simulink model "dvanaestaNedeljaPrimeri"  (R2018a)
settings: Solver=ode4  StartTime=0.0  StopTime=10  FixedStep=.01  RelTol=1e-3
values from neighbouring files (symbols this model uses):
  co = 10    [konstante.m]
  cp = [0 2 8]    [konstante.m]
  m = 1    [konstante.m]
undefined symbols (not defined in the file or in its folder): b
libraries: simulink x1
settings Model: Creator=Teodor  LastModifiedBy=Teodor

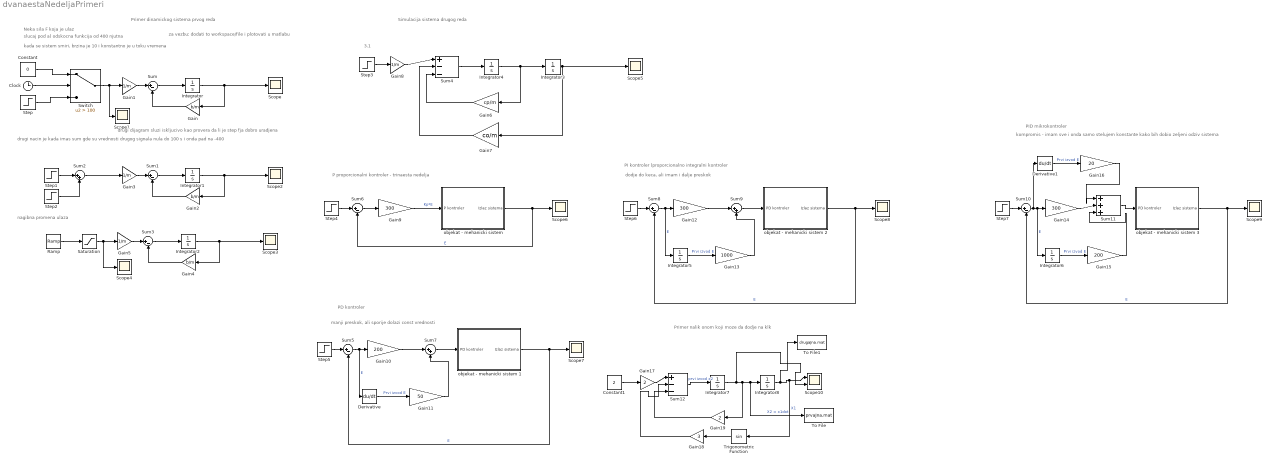
== system dvanaestaNedeljaPrimeri ==
  note: Primer nalik onom koji moze da dodje na klk
  note: kompromis - imam sve i onda samo stelujem konstante kako bih dobio zeljeni odziv sistema
  note: PID mikrokontroler
  note: dodje do keca, ali imam i dalje preskok
  note: PI kontroler (proporcionalno integralni kontroler
  note: manji preskok, ali sporije dolazi const vrednosti
  note: PD kontroler
  note: 3.1
  note: Simulacija sistema drugog reda
  note: za vezbu: dodati to workspace/file i plotovati u matlabu
  note: nagibna promena ulaza
  note: drugi nacin je kada imas sum gde su vrednosti drugog signala nula do 100 s i onda pad na -400
  note: kada se sistem smiri, brzina je 10 i konstantno je u toku vremena
  note: drugi dijagram sluzi iskljucivo kao provera da li je step fja dobro uradjena
  note: slucaj pod a) odskocna funkcija od 400 njutna
  note: Primer dinamickog sistema prvog reda
  note: Neka sila F koja je ulaz
  note: P proporcionalni kontroler - trinaesta nedelja
  Clock : Clock
  Constant : Constant  Value=0
  Constant1 : Constant  Value=2
  Derivative : Derivative
  Derivative1 : Derivative
  Gain : Gain  Gain=b/m
  Gain{1,3,5,8} (4 alike) : Gain  Gain=1/m
  Gain10 : Gain  Gain=200
  Gain11 : Gain  Gain=50
  Gain12 : Gain  Gain=300
  Gain13 : Gain  Gain=1000
  Gain14 : Gain  Gain=300
  Gain15 : Gain  Gain=200
  Gain16 : Gain  Gain=20
  Gain17 : Gain  Gain=2
  Gain18 : Gain  Gain=3
  Gain19 : Gain  Gain=2
  Gain2 : Gain  Gain=b/m
  Gain4 : Gain  Gain=b/m
  Gain6 : Gain  Gain=cp/m
  Gain7 : Gain  Gain=co/m
  Gain9 : Gain  Gain=300
  Integrator{,1..8} (9 alike) : Integrator
  Ramp : simulink/Sources/Ramp  slope=80  start=0  InitialOutput=0
  Saturation : Saturate  UpperLimit=2000  LowerLimit=0
  Scope{,1..9} (10 alike) : Scope
  Scope10 : Scope  NumInputPorts=2
  Step : Step  Time=0  After=400  SampleTime=0
  Step1 : Step  Time=0  After=400  SampleTime=0
  Step2 : Step  Time=100  After=-400  SampleTime=0
  Step3 : Step  Time=0  After=100  SampleTime=0
  Step{4..7} (4 alike) : Step  Time=0  SampleTime=0
  Sum{,1,3,5..6,8,10} (7 alike) : Sum  Inputs=|+-
  Sum11 : Sum  Inputs=|+++
  Sum12 : Sum  Inputs=|+--
  Sum2 : Sum  Inputs=|++
  Sum4 : Sum  Inputs=|+--
  Sum7 : Sum  Inputs=|++
  Sum9 : Sum  Inputs=|++
  Switch : Switch  Criteria=u2 > Threshold  Threshold=100
  To File : ToFile  Filename=prvaJna.mat  MatrixName=x2
  To File1 : ToFile  Filename=drugaJna.mat  MatrixName=x1
  Trigonometric Function : Trigonometry
  "objekat - mehanicki sistem " : Subsystem
  objekat - mehanicki sistem 1 : Subsystem
  objekat - mehanicki sistem 2 : Subsystem
  objekat - mehanicki sistem 3 : Subsystem
  wires:
  Sum/1 -> Integrator/1
  Gain1/1 -> Sum/1
  Integrator/1 -> Gain/1, Scope/1
  Gain/1 -> Sum/2
  Clock/1 -> Switch/2
  Switch/1 -> Scope1/1, Gain1/1
  Step/1 -> Switch/3
  Constant/1 -> Switch/1
  Gain2/1 -> Sum1/2
  Gain3/1 -> Sum1/1
  Sum1/1 -> Integrator1/1
  Sum2/1 -> Gain3/1
  Integrator1/1 -> Gain2/1, Scope2/1
  Step2/1 -> Sum2/2
  Step1/1 -> Sum2/1
  Sum3/1 -> Integrator2/1
  Gain4/1 -> Sum3/2
  Gain5/1 -> Sum3/1
  Integrator2/1 -> Gain4/1, Scope3/1
  Ramp/1 -> Saturation/1
  Saturation/1 -> Scope4/1, Gain5/1
  Integrator3/1 -> Gain7/1, Scope5/1
  Integrator4/1 -> Gain6/1, Integrator3/1
  Gain7/1 -> Sum4/2
  Gain6/1 -> Sum4/3
  Sum4/1 -> Integrator4/1
  Gain8/1 -> Sum4/1
  Step3/1 -> Gain8/1
  Step4/1 -> Sum6/1
  "objekat - mehanicki sistem "/1(Izlaz sistema) -> Scope6/1, Sum6/2  "E"
  Gain9/1 -> "objekat - mehanicki sistem "/1(P kontroler)  "Kp*E"
  Sum6/1 -> Gain9/1
  Step5/1 -> Sum5/1
  objekat - mehanicki sistem 1/1(Izlaz sistema) -> Scope7/1, Sum5/2  "E"
  Sum5/1 -> Derivative/1, Gain10/1  "E"
  Gain10/1 -> Sum7/1
  Derivative/1 -> Gain11/1  "Prvi izvod E"
  Gain11/1 -> Sum7/2
  Sum7/1 -> objekat - mehanicki sistem 1/1(PD kontroler)
  Gain12/1 -> Sum9/1
  Sum8/1 -> Integrator5/1, Gain12/1  "E"
  Integrator5/1 -> Gain13/1  "Prvi izvod E"
  Step6/1 -> Sum8/1
  Sum9/1 -> objekat - mehanicki sistem 2/1(PD kontroler)
  Gain13/1 -> Sum9/2
  objekat - mehanicki sistem 2/1(Izlaz sistema) -> Scope8/1, Sum8/2  "E"
  objekat - mehanicki sistem 3/1(Izlaz sistema) -> Scope9/1, Sum10/2  "E"
  Step7/1 -> Sum10/1
  Gain15/1 -> Sum11/3
  Sum11/1 -> objekat - mehanicki sistem 3/1(PD kontroler)
  Sum10/1 -> Derivative1/1, Integrator6/1, Gain14/1  "E"
  Gain14/1 -> Sum11/2
  Integrator6/1 -> Gain15/1  "Prvi izvod E"
  Derivative1/1 -> Gain16/1  "Prvi izvod E"
  Gain16/1 -> Sum11/1
  Constant1/1 -> Gain17/1
  Gain17/1 -> Sum12/1
  Sum12/1 -> Integrator7/1  "prvi izvod x2"
  Integrator8/1 -> To File1/1, Trigonometric Function/1, Scope10/1  "X1"
  Integrator7/1 -> Scope10/2, Gain19/1, To File/1, Integrator8/1  "X2 = x1dot"
  Trigonometric Function/1 -> Gain18/1
  Gain18/1 -> Sum12/2
  Gain19/1 -> Sum12/3

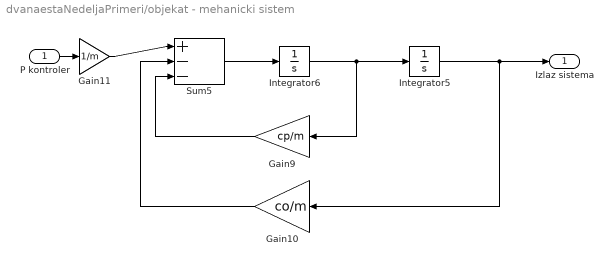
== system dvanaestaNedeljaPrimeri/objekat - mehanicki sistem  ==
  P kontroler : Inport
  Gain10 : Gain  Gain=co/m
  Gain11 : Gain  Gain=1/m
  Gain9 : Gain  Gain=cp/m
  Integrator5 : Integrator
  Integrator6 : Integrator
  Sum5 : Sum  Inputs=|+--
  Izlaz sistema : Outport
  wires:
  Sum5/1 -> Integrator6/1
  Gain11/1 -> Sum5/1
  Integrator6/1 -> Gain9/1, Integrator5/1
  Integrator5/1 -> Izlaz sistema/1, Gain10/1
  Gain9/1 -> Sum5/3
  Gain10/1 -> Sum5/2
  P kontroler/1 -> Gain11/1

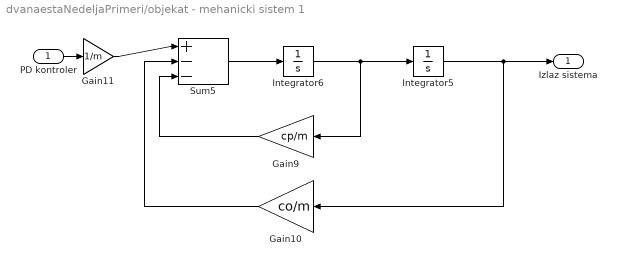
== system dvanaestaNedeljaPrimeri/objekat - mehanicki sistem 1 ==
  PD kontroler : Inport
  Gain10 : Gain  Gain=co/m
  Gain11 : Gain  Gain=1/m
  Gain9 : Gain  Gain=cp/m
  Integrator5 : Integrator
  Integrator6 : Integrator
  Sum5 : Sum  Inputs=|+--
  Izlaz sistema : Outport
  wires:
  Sum5/1 -> Integrator6/1
  Gain11/1 -> Sum5/1
  Integrator6/1 -> Gain9/1, Integrator5/1
  Integrator5/1 -> Izlaz sistema/1, Gain10/1
  Gain9/1 -> Sum5/3
  Gain10/1 -> Sum5/2
  PD kontroler/1 -> Gain11/1

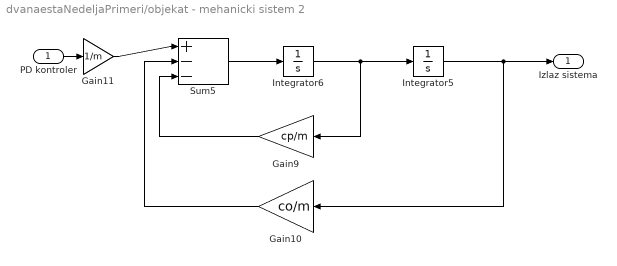
== system dvanaestaNedeljaPrimeri/objekat - mehanicki sistem 2 ==
  PD kontroler : Inport
  Gain10 : Gain  Gain=co/m
  Gain11 : Gain  Gain=1/m
  Gain9 : Gain  Gain=cp/m
  Integrator5 : Integrator
  Integrator6 : Integrator
  Sum5 : Sum  Inputs=|+--
  Izlaz sistema : Outport
  wires:
  Sum5/1 -> Integrator6/1
  Gain11/1 -> Sum5/1
  Integrator6/1 -> Gain9/1, Integrator5/1
  Integrator5/1 -> Izlaz sistema/1, Gain10/1
  Gain9/1 -> Sum5/3
  Gain10/1 -> Sum5/2
  PD kontroler/1 -> Gain11/1

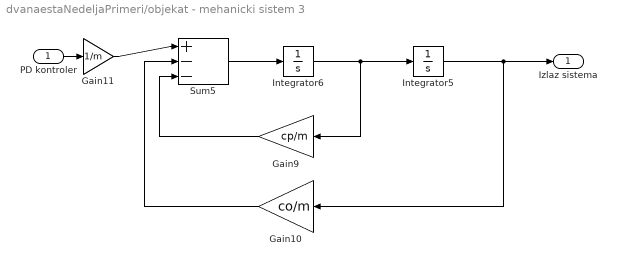
== system dvanaestaNedeljaPrimeri/objekat - mehanicki sistem 3 ==
  PD kontroler : Inport
  Gain10 : Gain  Gain=co/m
  Gain11 : Gain  Gain=1/m
  Gain9 : Gain  Gain=cp/m
  Integrator5 : Integrator
  Integrator6 : Integrator
  Sum5 : Sum  Inputs=|+--
  Izlaz sistema : Outport
  wires:
  Sum5/1 -> Integrator6/1
  Gain11/1 -> Sum5/1
  Integrator6/1 -> Gain9/1, Integrator5/1
  Integrator5/1 -> Izlaz sistema/1, Gain10/1
  Gain9/1 -> Sum5/3
  Gain10/1 -> Sum5/2
  PD kontroler/1 -> Gain11/1
